simulink model "trial2"  (R2021a)
settings: Solver=VariableStepAuto  StartTime=0.0  StopTime=10.0  RelTol=1e-3
settings Model: Creator=Aashish Kalra  LastModifiedBy=Aashish Kalra

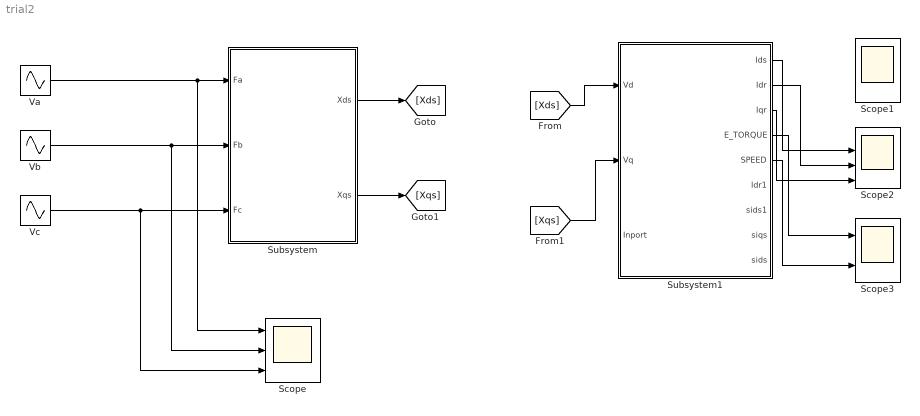
== system trial2 ==
  Scope : Scope  NumInputPorts=3
  Scope1 : Scope  NumInputPorts=2
  Scope2 : Scope  NumInputPorts=4
  Scope3 : Scope  NumInputPorts=2
  Subsystem : Subsystem
  Subsystem1 : Subsystem
  Va : Sin  Amplitude=200*sqrt(2)  Frequency=2*pi*50  Phase=((-2*pi)/3)+(pi/2)  SampleTime=0
  Vb : Sin  Amplitude=200*sqrt(2)  Frequency=2*pi*50  Phase=(pi/2)  SampleTime=0
  Vc : Sin  Amplitude=200*sqrt(2)  Frequency=2*pi*50  Phase=((2*pi)/3)+(pi/2)  SampleTime=0
  wires:
  Subsystem1/4("E_TORQUE ") -> Scope3/1
  Subsystem1/1(Ids) -> Scope2/2
  ? -> Scope1/1
  [Xds] -> Subsystem1/1(Vd)
  Subsystem1/5(SPEED) -> Scope3/2
  [Xqs] -> Subsystem1/2(Vq)
  ? -> Scope2/1
  Subsystem1/2(Idr) -> Scope2/3
  Vb/1 -> Scope/2, Subsystem/2(Fb)
  ? -> Scope1/2
  Subsystem1/3(Iqr) -> Scope2/4
  Va/1 -> Scope/1, Subsystem/1(Fa)
  Subsystem/2(Xqs) -> [Xqs]
  Subsystem/1(Xds) -> [Xds]
  Vc/1 -> Scope/3, Subsystem/3(Fc)

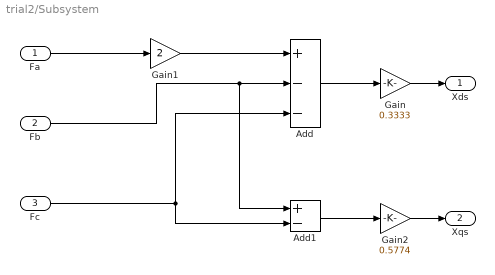
== system trial2/Subsystem ==
  Fa : Inport
  Fb : Inport  Port=2
  Fc : Inport  Port=3
  Add : Sum  Inputs=+--
  Add1 : Sum  Inputs=+-
  Gain : Gain  Gain=0.3333
  Gain1 : Gain  Gain=2
  Gain2 : Gain  Gain=0.5774
  Xds : Outport  VectorParamsAs1DForOutWhenUnconnected=off
  Xqs : Outport  Port=2  VectorParamsAs1DForOutWhenUnconnected=off
  wires:
  Fa/1 -> Gain1/1
  Gain/1 -> Xds/1
  Add/1 -> Gain/1
  Gain1/1 -> Add/1
  Fb/1 -> Add1/1, Add/2
  Fc/1 -> Add1/2, Add/3
  Add1/1 -> Gain2/1
  Gain2/1 -> Xqs/1

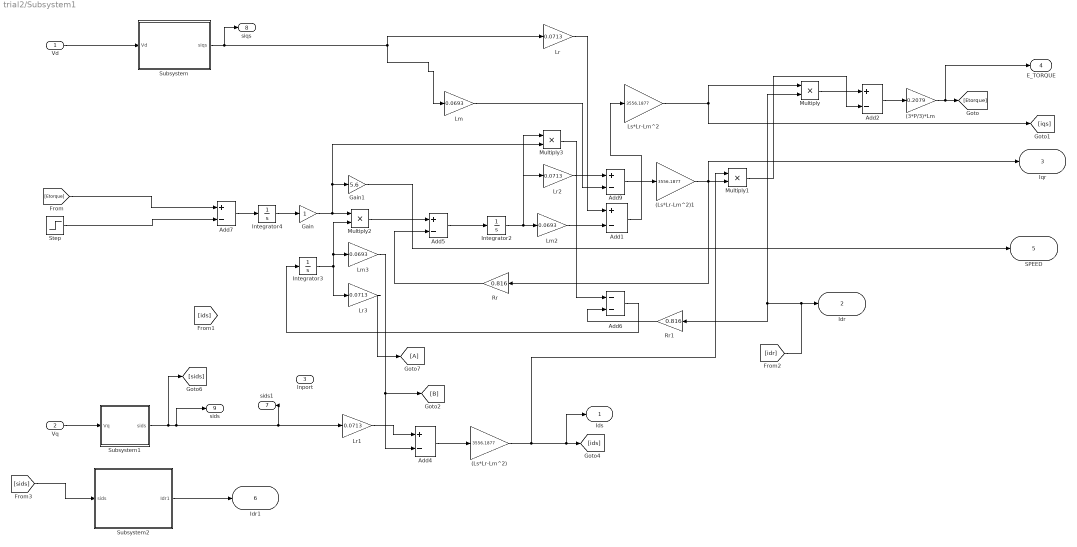
== system trial2/Subsystem1 ==
  Vd : Inport
  Vq : Inport  Port=2
  Inport : Inport  Port=3
  (3*P/3)*Lm : Gain  Gain=0.2079
  (Ls*Lr-Lm^2) : Gain  Gain=3556.1877
  (Ls*Lr-Lm^2)1 : Gain  Gain=3556.1877
  Add{1..2,4..5,7,9} (6 alike) : Sum  Inputs=+-
  Add6 : Sum  Inputs=--
  Gain : Gain
  Gain1 : Gain  Gain=5.6
  Integrator2 : Integrator
  Integrator3 : Integrator
  Integrator4 : Integrator
  Lm : Gain  Gain=0.0693
  Lm2 : Gain  Gain=0.0693
  Lm3 : Gain  Gain=0.0693
  Lr{,1..3} (4 alike) : Gain  Gain=0.0713
  Ls*Lr-Lm^2 : Gain  Gain=3556.1877
  Multiply{,1..3} (4 alike) : Product
  Rr : Gain  Gain=0.816
  Rr1 : Gain  Gain=0.816
  Step : Step  Time=5  After=20  SampleTime=0
  Subsystem : Subsystem
  Subsystem1 : Subsystem
  Subsystem2 : Subsystem
  Ids : Outport  VectorParamsAs1DForOutWhenUnconnected=off
  Idr : Outport  Port=2  VectorParamsAs1DForOutWhenUnconnected=off
  Iqr : Outport  Port=3  VectorParamsAs1DForOutWhenUnconnected=off
  "E_TORQUE " : Outport  Port=4  VectorParamsAs1DForOutWhenUnconnected=off
  SPEED : Outport  Port=5  VectorParamsAs1DForOutWhenUnconnected=off
  Idr1 : Outport  Port=6  VectorParamsAs1DForOutWhenUnconnected=off
  sids1 : Outport  Port=7  VectorParamsAs1DForOutWhenUnconnected=off
  siqs : Outport  Port=8
  sids : Outport  Port=9
  wires:
  (3*P/3)*Lm/1 -> [Etorque], "E_TORQUE "/1
  Add6/1 -> Integrator3/1
  Rr/1 -> Add5/2
  Multiply2/1 -> Add5/1
  Lr/1 -> Add1/1
  Add9/1 -> (Ls*Lr-Lm^2)1/1
  Add5/1 -> Integrator2/1
  Lm3/1 -> Add4/2, [B]
  Ls*Lr-Lm^2/1 -> [iqs], Multiply/1
  Multiply/1 -> Add2/1
  Multiply3/1 -> Add6/1
  Add1/1 -> Ls*Lr-Lm^2/1
  Rr1/1 -> Add6/2
  [Etorque] -> Add7/1
  Add7/1 -> Integrator4/1
  Lr3/1 -> [A]
  Integrator2/1 -> Lr2/1, Lm2/1, Multiply3/1
  Lm/1 -> Add9/2
  Lm2/1 -> Add1/2
  (Ls*Lr-Lm^2)1/1 -> Multiply1/2, Iqr/1, Rr/1
  (Ls*Lr-Lm^2)/1 -> Multiply1/1, Ids/1, [ids]
  Multiply1/1 -> Add2/2
  Integrator3/1 -> Lr3/1, Multiply2/2, Lm3/1
  Step/1 -> Add7/2
  Add2/1 -> (3*P/3)*Lm/1
  Gain1/1 -> SPEED/1
  Add4/1 -> (Ls*Lr-Lm^2)/1
  Gain/1 -> Gain1/1, Multiply3/2, Multiply2/1
  Lr1/1 -> Add4/1
  Lr2/1 -> Add9/1
  Integrator4/1 -> Gain/1
  Subsystem/1(siqs) -> siqs/1, Lm/1, Lr/1
  Vd/1 -> Subsystem/1(Vd)
  Subsystem1/1(sids) -> [sids], sids/1, sids1/1, Lr1/1
  Vq/1 -> Subsystem1/1(Vq)
  [idr] -> Rr1/1, Multiply/2, Idr/1
  Subsystem2/1(Idr1) -> Idr1/1
  [sids] -> Subsystem2/1(sids)

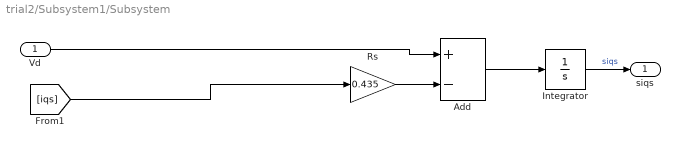
== system trial2/Subsystem1/Subsystem ==
  Vd : Inport
  Add : Sum  Inputs=+-
  Integrator : Integrator
  Rs : Gain  Gain=0.435
  siqs : Outport
  wires:
  Add/1 -> Integrator/1
  [iqs] -> Rs/1
  Vd/1 -> Add/1
  Rs/1 -> Add/2
  Integrator/1 -> siqs/1  "siqs"

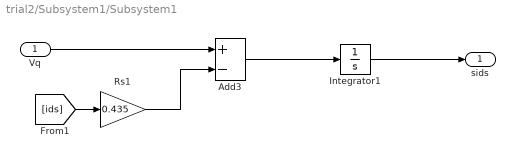
== system trial2/Subsystem1/Subsystem1 ==
  Vq : Inport
  Add3 : Sum  Inputs=+-
  Integrator1 : Integrator
  Rs1 : Gain  Gain=0.435
  sids : Outport  VectorParamsAs1DForOutWhenUnconnected=off
  wires:
  Integrator1/1 -> sids/1
  [ids] -> Rs1/1
  Rs1/1 -> Add3/2
  Vq/1 -> Add3/1
  Add3/1 -> Integrator1/1

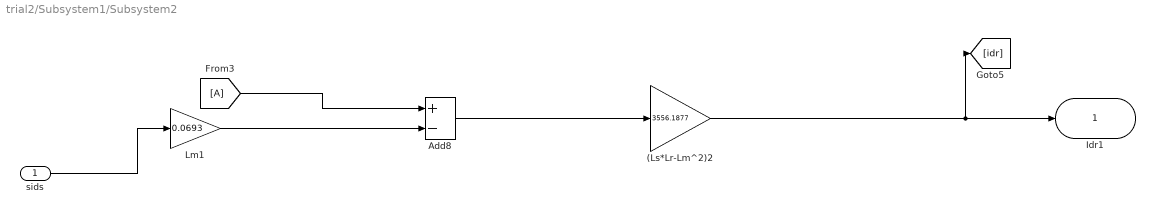
== system trial2/Subsystem1/Subsystem2 ==
  sids : Inport
  (Ls*Lr-Lm^2)2 : Gain  Gain=3556.1877
  Add8 : Sum  Inputs=+-
  Lm1 : Gain  Gain=0.0693
  Idr1 : Outport  VectorParamsAs1DForOutWhenUnconnected=off
  wires:
  [A] -> Add8/1
  Lm1/1 -> Add8/2
  (Ls*Lr-Lm^2)2/1 -> Idr1/1, [idr]
  Add8/1 -> (Ls*Lr-Lm^2)2/1
  sids/1 -> Lm1/1
